simulink library "HORTISIM"  (R2021a)
settings: Solver=VariableStepAuto  StartTime=0.0  StopTime=10.0  RelTol=1e-3
undefined symbols (not defined in the file or in its folder): crop_params, heat_ic, heat_p, p_climate, params_fruit, scr_p, substrate_params, tp_tilapia, win_p, x0_climate, x0_crop, x0_fruit, x0_substrate, x0_tank_tilapia
libraries: $bdroot x10
(part 4 of 4)

== system HORTISIM/Horticulture/Models/Crop Grow/Crop Growth/Growth model/Respiration ==
  T_vmean : Inport
  Crop : Inport  Port=2
  MC_gro : Inport  Port=3
  Bus Creator : BusCreator  Inputs=4
  Bus Selector : BusSelector  OutputSignals=Carbon.Cfruit,Relative.Rfruit,Carbon.Cleaf,Relative.Rleaf,Carbon.Cstem,Relative.Rstem
  Bus Selector2 : BusSelector  OutputSignals=MC_buf_fruit,MC_buf_leaf,MC_buf_stem
  Constant : Constant  Value=params.c_fruit_g
  Constant1 : Constant  Value=params.c_leaf_g
  Constant2 : Constant  Value=params.c_stem_g
  Constant3 : Constant  Value=params.c_fruit_m
  Constant4 : Constant  Value=params.c_leaf_m
  Constant5 : Constant  Value=params.c_stem_m
  Product : Product
  Product1 : Product
  Product2 : Product
  Scope : Scope  NumInputPorts=4
  Subsystem : Subsystem
      settings: PortSchema="{\"entries\":[{\"content\":{\"sides\":[{\"content\":{\"connectorIds\":[\"In1\",\"In2\",\"In3\"]},\"type\":\"ConnectorPlacement.EquallySpacedRectSide\",\"uuid\":\"e383cf86-92c2-4a3a-a03f-0f03c9e6b06e\"},{\"content\":{\"connectorIds\":[\"Out1\"],\"side\":\"RIGHT\"},\"type\":\"ConnectorPlacement.EquallySpacedRectSide\",\"uuid\":\"c4c6234d-4969-4652-ba5e-e62d60415ae5\"},{\"content\":{\"connectorIds\":[\"In4\"],\"side\":\"TOP\"},\"type\":\"ConnectorPlacement.EquallySpacedRectSide\",\"uuid\":\"e372fef3-870c-4656-925c-98a7f16866f7\"}]},\"type\":\"ConnectorPlacement.EquallySpacedConnector\",\"uuid\":\"336e0ef1-3fb5-46ea-bbca-17f64dad2455\"}],\"packageUris\":[\"http://schema.mathworks.com/mf0/Connector/R2020b\"],\"version\":\"1.0\"}"
  Subsystem1 : Subsystem
      settings: PortSchema="{\"entries\":[{\"content\":{\"sides\":[{\"content\":{\"connectorIds\":[\"In1\",\"In2\",\"In3\"]},\"type\":\"ConnectorPlacement.EquallySpacedRectSide\",\"uuid\":\"e383cf86-92c2-4a3a-a03f-0f03c9e6b06e\"},{\"content\":{\"connectorIds\":[\"Out1\"],\"side\":\"RIGHT\"},\"type\":\"ConnectorPlacement.EquallySpacedRectSide\",\"uuid\":\"c4c6234d-4969-4652-ba5e-e62d60415ae5\"},{\"content\":{\"connectorIds\":[\"In4\"],\"side\":\"TOP\"},\"type\":\"ConnectorPlacement.EquallySpacedRectSide\",\"uuid\":\"e372fef3-870c-4656-925c-98a7f16866f7\"}]},\"type\":\"ConnectorPlacement.EquallySpacedConnector\",\"uuid\":\"336e0ef1-3fb5-46ea-bbca-17f64dad2455\"}],\"packageUris\":[\"http://schema.mathworks.com/mf0/Connector/R2020b\"],\"version\":\"1.0\"}"
  Subsystem2 : Subsystem
      settings: PortSchema="{\"entries\":[{\"content\":{\"sides\":[{\"content\":{\"connectorIds\":[\"In1\",\"In2\",\"In3\"]},\"type\":\"ConnectorPlacement.EquallySpacedRectSide\",\"uuid\":\"e383cf86-92c2-4a3a-a03f-0f03c9e6b06e\"},{\"content\":{\"connectorIds\":[\"Out1\"],\"side\":\"RIGHT\"},\"type\":\"ConnectorPlacement.EquallySpacedRectSide\",\"uuid\":\"c4c6234d-4969-4652-ba5e-e62d60415ae5\"},{\"content\":{\"connectorIds\":[\"In4\"],\"side\":\"TOP\"},\"type\":\"ConnectorPlacement.EquallySpacedRectSide\",\"uuid\":\"e372fef3-870c-4656-925c-98a7f16866f7\"}]},\"type\":\"ConnectorPlacement.EquallySpacedConnector\",\"uuid\":\"336e0ef1-3fb5-46ea-bbca-17f64dad2455\"}],\"packageUris\":[\"http://schema.mathworks.com/mf0/Connector/R2020b\"],\"version\":\"1.0\"}"
  Sum : Sum  Inputs=|+++
  MC_resp : Outport
  wires:
  Constant5/1 -> Subsystem2/3(c_m)
  Constant4/1 -> Subsystem1/3(c_m)
  [T_v] -> Subsystem2/4(T_vmean)
  [T_v] -> Subsystem1/4(T_vmean)
  [T_v] -> Subsystem/4(T_vmean)
  Constant3/1 -> Subsystem/3(c_m)
  T_vmean/1 -> [T_v]
  Product1/1 -> Sum/3
  Product2/1 -> Sum/2
  Constant1/1 -> Product2/2
  Constant/1 -> Product/2
  Constant2/1 -> Product1/2
  Product/1 -> Sum/1
  Sum/1 -> Scope/1, Bus Creator/1  "MC_buf_i"
  Bus Selector2/3 -> Product1/1  "<MC_buf_stem>"
  Bus Selector2/2 -> Product2/1  "<MC_buf_leaf>"
  Bus Selector2/1 -> Product/1  "<MC_buf_fruit>"
  Bus Creator/1 -> MC_resp/1
  Subsystem/1(MC_fruit_i) -> Scope/4, Bus Creator/2  "MC_fruit_i"
  Subsystem1/1(MC_leaf_i) -> Scope/2, Bus Creator/3  "MC_leaf_i"
  Subsystem2/1(MC_steam_i) -> Scope/3, Bus Creator/4  "MC_stem_i"
  MC_gro/1 -> Bus Selector2/1
  Crop/1 -> Bus Selector/1
  Bus Selector/1 -> Subsystem/1(C)  "<Cfruit>"
  Bus Selector/2 -> Subsystem/2(R)  "<Rfruit>"
  Bus Selector/3 -> Subsystem1/1(C)  "<Cleaf>"
  Bus Selector/4 -> Subsystem1/2(R)  "<Rleaf>"
  Bus Selector/5 -> Subsystem2/1(C)  "<Cstem>"
  Bus Selector/6 -> Subsystem2/2(R)  "<Rstem>"

== system HORTISIM/Horticulture/Models/Crop Grow/Crop Growth/Growth model/Subsystem2 ==
  " " : Inport
  "         " : Inport  Port=2
  Bus Creator : BusCreator  Inputs=5
  Demux : Demux
  "   " : Outport
  wires:
  "         "/1 -> Demux/1
  Demux/2 -> Bus Creator/3  "MC_fruit_i"
  Demux/1 -> Bus Creator/2  "MC_buf_i"
  Demux/3 -> Bus Creator/4  "MC_leaf_i"
  " "/1 -> Bus Creator/1  "MC_i_buf"
  Bus Creator/1 -> "   "/1
  Demux/4 -> Bus Creator/5  "MC_stem_i"

== system HORTISIM/Horticulture/Models/Crop Grow/Merges/Subsystem/Convertion Ratio ==
  Constant : Constant
  Constant1 : Constant  Value=params.fraction_DM
  Divide : Product  Inputs=*/
  Minus : Sum  Inputs=+-
  Out1 : Outport
  wires:
  Minus/1 -> Out1/1
  Constant1/1 -> Divide/2
  Constant/1 -> Divide/1, Minus/2
  Divide/1 -> Minus/1

== system HORTISIM/Horticulture/Models/Substrate Bag/Subsystem3/V0/Subsystem ==
  V : Inport
  Constant : Constant  Value=params.Vmax_subs/3
  Constant1 : Constant  Value=0.5
  Gain : Gain  Gain=500
  Gain3 : Gain  Gain=0.5
  Minus1 : Sum  Inputs=+-
  Product : Product
  Sum1 : Sum  Inputs=|++
  Tanh : Trigonometry  Operator=tanh
  Out1 : Outport
  wires:
  Tanh/1 -> Gain3/1
  Constant1/1 -> Sum1/2
  Gain3/1 -> Sum1/1
  Gain/1 -> Tanh/1
  Constant/1 -> Minus1/2
  V/1 -> Minus1/1
  Minus1/1 -> Product/1, Gain/1
  Sum1/1 -> Product/2
  Product/1 -> Out1/1

== system HORTISIM/Horticulture/Models/Substrate Bag/Subsystem3/V0/Subsystem1 ==
  V : Inport
  Constant1 : Constant  Value=0.5
  Constant2 : Constant  Value=params.Vmin_subs/3
  Gain : Gain  Gain=5e4
  Gain3 : Gain  Gain=0.5
  Minus1 : Sum  Inputs=+-
  Sum1 : Sum  Inputs=|++
  Tanh : Trigonometry  Operator=tanh
  Out1 : Outport
  wires:
  Tanh/1 -> Gain3/1
  Sum1/1 -> Out1/1
  Constant1/1 -> Sum1/2
  Gain3/1 -> Sum1/1
  Gain/1 -> Tanh/1
  Constant2/1 -> Minus1/2
  V/1 -> Minus1/1
  Minus1/1 -> Gain/1

== system HORTISIM/Horticulture/Models/Substrate Bag/Subsystem3/V1/Subsystem ==
  V : Inport
  Constant : Constant  Value=params.Vmax_subs/3
  Constant1 : Constant  Value=0.5
  Gain : Gain  Gain=500
  Gain3 : Gain  Gain=0.5
  Minus1 : Sum  Inputs=+-
  Product : Product
  Sum1 : Sum  Inputs=|++
  Tanh : Trigonometry  Operator=tanh
  Out1 : Outport
  wires:
  Tanh/1 -> Gain3/1
  Constant1/1 -> Sum1/2
  Gain3/1 -> Sum1/1
  Gain/1 -> Tanh/1
  Constant/1 -> Minus1/2
  V/1 -> Minus1/1
  Minus1/1 -> Product/1, Gain/1
  Sum1/1 -> Product/2
  Product/1 -> Out1/1

== system HORTISIM/Horticulture/Models/Substrate Bag/Subsystem3/V1/Subsystem1 ==
  V : Inport
  Constant1 : Constant  Value=0.5
  Constant2 : Constant  Value=params.Vmin_subs/3
  Gain : Gain  Gain=5e4
  Gain3 : Gain  Gain=0.5
  Minus1 : Sum  Inputs=+-
  Sum1 : Sum  Inputs=|++
  Tanh : Trigonometry  Operator=tanh
  Out1 : Outport
  wires:
  Tanh/1 -> Gain3/1
  Sum1/1 -> Out1/1
  Constant1/1 -> Sum1/2
  Gain3/1 -> Sum1/1
  Gain/1 -> Tanh/1
  Constant2/1 -> Minus1/2
  V/1 -> Minus1/1
  Minus1/1 -> Gain/1

== system HORTISIM/Horticulture/Models/Substrate Bag/Subsystem3/V2/Subsystem ==
  V : Inport
  Constant : Constant  Value=params.Vmax_subs/3
  Constant1 : Constant  Value=0.5
  Gain : Gain  Gain=500
  Gain3 : Gain  Gain=0.5
  Minus1 : Sum  Inputs=+-
  Product : Product
  Sum1 : Sum  Inputs=|++
  Tanh : Trigonometry  Operator=tanh
  Out1 : Outport
  wires:
  Tanh/1 -> Gain3/1
  Constant1/1 -> Sum1/2
  Gain3/1 -> Sum1/1
  Gain/1 -> Tanh/1
  Constant/1 -> Minus1/2
  V/1 -> Minus1/1
  Minus1/1 -> Product/1, Gain/1
  Sum1/1 -> Product/2
  Product/1 -> Out1/1

== system HORTISIM/Horticulture/Models/Substrate Bag/Subsystem3/V2/Subsystem1 ==
  V : Inport
  Constant1 : Constant  Value=0.5
  Constant2 : Constant  Value=params.Vmin_subs/3
  Gain : Gain  Gain=5e4
  Gain3 : Gain  Gain=0.5
  Minus1 : Sum  Inputs=+-
  Sum1 : Sum  Inputs=|++
  Tanh : Trigonometry  Operator=tanh
  Out1 : Outport
  wires:
  Tanh/1 -> Gain3/1
  Sum1/1 -> Out1/1
  Constant1/1 -> Sum1/2
  Gain3/1 -> Sum1/1
  Gain/1 -> Tanh/1
  Constant2/1 -> Minus1/2
  V/1 -> Minus1/1
  Minus1/1 -> Gain/1

== system HORTISIM/Aquaculture/Models/Tank Model/Heat Balances/Convection Air 2 Water Tanl Surface/Gr2vG/If Action Subsystem ==
  Gr : Inport
  Action Port : ActionPort
  Constant : Constant  Value=0.25
  Gain : Gain  Gain=0.5
  Pow : Math  Operator=pow  SignedPower=on  RndMeth=Zero  SaturateOnIntegerOverflow=on
  Out1 : Outport
  wires:
  Gr/1 -> Pow/1
  Constant/1 -> Pow/2
  Pow/1 -> Gain/1
  Gain/1 -> Out1/1

== system HORTISIM/Aquaculture/Models/Tank Model/Heat Balances/Convection Air 2 Water Tanl Surface/Gr2vG/If Action Subsystem1 ==
  Gr : Inport
  Action Port : ActionPort
  Constant : Constant  Value=0.25
  Gain : Gain  Gain=0.5
  Pow : Math  Operator=pow  SignedPower=on  RndMeth=Zero  SaturateOnIntegerOverflow=on
  Out1 : Outport
  wires:
  Gain/1 -> Out1/1
  Constant/1 -> Pow/2
  Gr/1 -> Pow/1
  Pow/1 -> Gain/1

== system HORTISIM/Aquaculture/Models/Tank Model/Heat Balances/Convection Air 2 Water Tanl Surface/Re2vR/If Action Subsystem ==
  Re : Inport
  Action Port : ActionPort
  Constant : Constant  Value=0.5
  Gain : Gain  Gain=0.6
  Pow : Math  Operator=pow  SignedPower=on  RndMeth=Zero  SaturateOnIntegerOverflow=on
  Out1 : Outport
  wires:
  Re/1 -> Pow/1
  Constant/1 -> Pow/2
  Pow/1 -> Gain/1
  Gain/1 -> Out1/1

== system HORTISIM/Aquaculture/Models/Tank Model/Heat Balances/Convection Air 2 Water Tanl Surface/Re2vR/If Action Subsystem1 ==
  Re : Inport
  Action Port : ActionPort
  Constant : Constant  Value=0.8
  Gain : Gain  Gain=0.032
  Pow : Math  Operator=pow  SignedPower=on  RndMeth=Zero  SaturateOnIntegerOverflow=on
  Out1 : Outport
  wires:
  Gain/1 -> Out1/1
  Constant/1 -> Pow/2
  Re/1 -> Pow/1
  Pow/1 -> Gain/1

== system HORTISIM/Aquaculture/Models/Tank Model/Heat Balances/Convection Air 2 Water Tanl Surface/Subsystem/If Action Subsystem ==
  In1 : Inport
  In2 : Inport  Port=2
  Action Port : ActionPort
  Out1 : Outport
  Out2 : Outport  Port=2
  wires:
  In1/1 -> Out1/1
  In2/1 -> Out2/1

== system HORTISIM/Aquaculture/Models/Tank Model/Heat Balances/Convection Air 2 Water Tanl Surface/Subsystem/If Action Subsystem1 ==
  In1 : Inport
  In2 : Inport  Port=2
  Action Port : ActionPort
  Out1 : Outport
  Out2 : Outport  Port=2
  wires:
  In1/1 -> Out1/1
  In2/1 -> Out2/1

== system HORTISIM/Aquaculture/Models/Tank Model/Subsystem/Subsystem1/For Each Subsystem/If Action Subsystem ==
  In1 : Inport
  Action Port : ActionPort
  Out1 : Outport
  wires:
  In1/1 -> Out1/1

== system HORTISIM/Aquaculture/Models/Tank Model/Subsystem/Subsystem1/For Each Subsystem/If Action Subsystem1 ==
  X : Inport
  Action Port : ActionPort
  Out1 : Outport
  wires:
  X/1 -> Out1/1

== system HORTISIM/Climate/Models/Climate Model/Gases Exchange/Compute Mid Variables/Subsystem/Ratio of Humidity Sat ==
  <Tair> : Inport
  p_a : Inport  Port=2
  sat_C_w : Inport  Port=3
  " molar mass of water [kg/mol]" : Constant  Value=0.0180
  Divide1 : Product  Inputs=*/
  Divide2 : Product  Inputs=*/
  Gain1 : Gain  Gain=0.62198
  Minus : Sum  Inputs=+-
  Product : Product  Inputs=3
  gas constant [J/mol/K] : Constant  Value=8.3140
  Out1 : Outport
  wires:
  p_a/1 -> Minus/1
  Minus/1 -> Divide2/2
  Gain1/1 -> Out1/1
  sat_C_w/1 -> Product/3
  <Tair>/1 -> Product/1
  Product/1 -> Divide1/1
  " molar mass of water [kg/mol]"/1 -> Divide1/2
  gas constant [J/mol/K]/1 -> Product/2
  Divide1/1 -> Divide2/1, Minus/2  "p_w^*"
  Divide2/1 -> Gain1/1

== system HORTISIM/Horticulture/Models/Crop Grow/Crop Growth/Growth model/Respiration/Subsystem ==
  C : Inport
  R : Inport  Port=2
  c_m : Inport  Port=3
  T_vmean : Inport  Port=4
  Exponetial Term : Subsystem
  Gain : Gain  Gain=0.1
  Minus : Sum  Inputs=+-
  Power : Math  Operator=pow  SaturateOnIntegerOverflow=on
  Product2 : Product  Inputs=4
  Q_10 : Constant  Value=2
  T_25 : Constant  Value=298.1500
  MC_fruit_i : Outport
  wires:
  Product2/1 -> MC_fruit_i/1
  C/1 -> Product2/4
  c_m/1 -> Product2/3
  Power/1 -> Product2/2
  Q_10/1 -> Power/1
  Exponetial Term/1(Out1) -> Product2/1
  R/1 -> Exponetial Term/1(In1)
  Gain/1 -> Power/2
  Minus/1 -> Gain/1
  T_25/1 -> Minus/2
  T_vmean/1 -> Minus/1

== system HORTISIM/Horticulture/Models/Crop Grow/Crop Growth/Growth model/Respiration/Subsystem1 ==
  C : Inport
  R : Inport  Port=2
  c_m : Inport  Port=3
  T_vmean : Inport  Port=4
  Exponetial Term : Subsystem
  Gain : Gain  Gain=0.1
  Minus : Sum  Inputs=+-
  Power : Math  Operator=pow  SaturateOnIntegerOverflow=on
  Product2 : Product  Inputs=4
  Q_10 : Constant  Value=2
  T_25 : Constant  Value=298.1500
  MC_leaf_i : Outport
  wires:
  Product2/1 -> MC_leaf_i/1
  C/1 -> Product2/4
  c_m/1 -> Product2/3
  Power/1 -> Product2/2
  Q_10/1 -> Power/1
  Exponetial Term/1(Out1) -> Product2/1
  R/1 -> Exponetial Term/1(In1)
  Gain/1 -> Power/2
  Minus/1 -> Gain/1
  T_25/1 -> Minus/2
  T_vmean/1 -> Minus/1

== system HORTISIM/Horticulture/Models/Crop Grow/Crop Growth/Growth model/Respiration/Subsystem2 ==
  C : Inport
  R : Inport  Port=2
  c_m : Inport  Port=3
  T_vmean : Inport  Port=4
  Exponetial Term : Subsystem
  Gain : Gain  Gain=0.1
  Minus : Sum  Inputs=+-
  Power : Math  Operator=pow  SaturateOnIntegerOverflow=on
  Product2 : Product  Inputs=4
  Q_10 : Constant  Value=2
  T_25 : Constant  Value=298.1500
  MC_steam_i : Outport
  wires:
  Product2/1 -> MC_steam_i/1
  C/1 -> Product2/4
  c_m/1 -> Product2/3
  Power/1 -> Product2/2
  Q_10/1 -> Power/1
  Exponetial Term/1(Out1) -> Product2/1
  R/1 -> Exponetial Term/1(In1)
  Gain/1 -> Power/2
  Minus/1 -> Gain/1
  T_25/1 -> Minus/2
  T_vmean/1 -> Minus/1

== system HORTISIM/Horticulture/Models/Crop Grow/Crop Growth/Growth model/Respiration/Subsystem/Exponetial Term ==
  In1 : Inport
  Constant : Constant
  Exp : Math  SaturateOnIntegerOverflow=on
  Gain1 : Gain  Gain=-1
  Minus1 : Sum  Inputs=+-
  Product1 : Product
  regression coefficient in maintenance respiration function [s] : Constant  Value=2850000
  Out1 : Outport
  wires:
  Product1/1 -> Gain1/1
  Constant/1 -> Minus1/1
  Gain1/1 -> Exp/1
  Exp/1 -> Minus1/2
  regression coefficient in maintenance respiration function [s]/1 -> Product1/2
  Minus1/1 -> Out1/1
  In1/1 -> Product1/1

== system HORTISIM/Horticulture/Models/Crop Grow/Crop Growth/Growth model/Respiration/Subsystem1/Exponetial Term ==
  In1 : Inport
  Constant : Constant
  Exp : Math  SaturateOnIntegerOverflow=on
  Gain1 : Gain  Gain=-1
  Minus1 : Sum  Inputs=+-
  Product1 : Product
  regression coefficient in maintenance respiration function [s] : Constant  Value=2850000
  Out1 : Outport
  wires:
  Product1/1 -> Gain1/1
  Constant/1 -> Minus1/1
  Gain1/1 -> Exp/1
  Exp/1 -> Minus1/2
  regression coefficient in maintenance respiration function [s]/1 -> Product1/2
  Minus1/1 -> Out1/1
  In1/1 -> Product1/1

== system HORTISIM/Horticulture/Models/Crop Grow/Crop Growth/Growth model/Respiration/Subsystem2/Exponetial Term ==
  In1 : Inport
  Constant : Constant
  Exp : Math  SaturateOnIntegerOverflow=on
  Gain1 : Gain  Gain=-1
  Minus1 : Sum  Inputs=+-
  Product1 : Product
  regression coefficient in maintenance respiration function [s] : Constant  Value=2850000
  Out1 : Outport
  wires:
  Product1/1 -> Gain1/1
  Constant/1 -> Minus1/1
  Gain1/1 -> Exp/1
  Exp/1 -> Minus1/2
  regression coefficient in maintenance respiration function [s]/1 -> Product1/2
  Minus1/1 -> Out1/1
  In1/1 -> Product1/1

== matlab function HORTISIM/Climate/Models/Climate Model/Indoor Temperature Model/Conduction/Conduction ==
  data: T_f input; T_s1 input; QD_sf1 output; QD_s12 output; A_f input; lam_s input; l_s input; T_ss input
function [QD_sf1,QD_s12] = fcn(T_f,T_s1,A_f,lam_s,l_s,T_ss)

%
%%
% GEOMETRY
% ========
% A_f = p.A_f; % greenhouse floor area [m^2]
% 
% % FLOOR 
% % =====================
% lam_s= p.lam_s; %thermal conductivity of soil layers [W/mK] Concrete, Soil, Clay
% l_s  = p.l_s; %thickness of soil layers [m]
% 
% T_ss = p.T_ss; %deep soil temperature [K]

%%      Conduction
% Floor layers 
% 
QD_sf1 = A_f*lam_s(1)/l_s(1).*(T_f - T_s1); 
QD_s12 = A_f*lam_s(2)/l_s(2).*(T_s1 - T_ss);

== matlab function HORTISIM/Climate/Models/Climate Model/Indoor Temperature Model/Convection/Convection/Convection ==
  data: QV_c_e output; QV_i_c output; QV_i_f output; T_c input; T_i input; T_f input; T_e input; wind_speed input; QP_i_c output; QP_i_f output; C_w input; rho_i input; A_f input; A_c input; d_c input; d_f input; int_air_speed input; C_w_sat_T_c input; C_w_sat_T_f input
function [QV_c_e,QV_i_c,QV_i_f,QP_i_c,QP_i_f] = fcn( T_c,T_i,T_f,T_e,wind_speed,C_w,rho_i,A_f,A_c,d_c,d_f,int_air_speed,C_w_sat_T_c,C_w_sat_T_f)

% CONSTANTS
% =========
g = 9.8100; % acceleration due to gravity [m/s^2]
lambda = 0.0250; % thermal conductivity of air [W/m/K]

Le = 0.8190; % Lewis number [-] 
nu =  1.5100e-05; % kinematic viscosity [m^2/s]

%%
c_i = 1.0032e+03;
H_fg = 2437000;

%%

if wind_speed<0
    wind_speed = 0;
end
%%      Convection

% The Grashof and Reynolds numbers are calculated, and then the Nusselt
% number calculated as the larger of the 'free' Nusselt number, based on
% the Grashof number, and the 'forced' Nusselt number, based on the
% Reynolds number. The heat transferred per unit time is then calculated
% based on this. The first subscript is where heat is transferred from, and
% the second subscript where heat is transferred to.

% Cover to external air
Gr = g*d_c^3/(T_e*nu^2)*abs(T_c - T_e);
Re = wind_speed*d_c/nu;
Nu = lamorturb(Gr, Re);
QV_c_e = 4*A_c.*Nu*lambda.*(T_c - T_e)/d_c;

% Internal air to cover
Gr = g*d_c^3./(T_i*nu^2).*abs(T_i - T_c);
Re = int_air_speed*d_c/nu;  
[Nu, Sh] = lamorturb(Gr, Re, Le);
QV_i_c = 4*A_c.*Nu*lambda.*(T_i - T_c)/d_c;
QP_i_c = 4*A_c*H_fg./(rho_i*c_i).*Sh/Le*lambda/d_c.*(C_w - C_w_sat_T_c);
%QP_i_c = max(QP_i_c,0); % assumed no evaporation from the cover, only condensation

%Internal air to floor
Gr = g*d_f^3./(T_i*nu^2).*abs(T_i - T_f); 
Re = int_air_speed*d_f/nu;
[Nu, Sh] = lamorturb(Gr, Re, Le);
QV_i_f = A_f.*Nu*lambda.*(T_i - T_f)/d_f;
QP_i_f = A_f*H_fg./(rho_i*c_i).*Sh/Le*lambda/d_f.*(C_w - C_w_sat_T_f); 
%QP_i_f = max(QP_i_f,0); % assumed no evaporation from the floor, only condensation

== matlab function HORTISIM/Horticulture/Models/Fruit Partitioning1/MATLAB Function ==
  data: Cfruit input; dCmdt output; Tsum input; Cfruit_mature input; T input; DT output
function [dCmdt,DT] = fcn(Cfruit, Tsum, Cfruit_mature,T)

a = 0.05;

T = T-273.15;
DT = a*max(0,min(1,0.0714*(T-9)));

dCmdt = (Tsum<2600)*DT*(Tsum>1200)*(Cfruit-Cfruit_mature);

== matlab function HORTISIM/Climate/Models/Climate Model/Indoor Temperature Model/Heat Balance/ Soil ==
  data: QD_sf1 input; QD_s12 input; dT_s1_dt output; A_f input; c_s input; l_s input; rhod_s input
function dT_s1_dt  = fcn(QD_sf1,QD_s12,A_f,c_s,l_s,rhod_s)



%% Soil 1
c_Ts1 = 1./(rhod_s(2) * c_s(2) * l_s(2)*A_f);
%
dT_s1_dt = c_Ts1*(QD_sf1 - QD_s12);
%%

== matlab function HORTISIM/Horticulture/Models/Crop Grow/Air Convection/ Temperature ==
  data: QS_v_VIS input; QT_v_i input; QV_v_i input; dT_v_dt output; A_v input; LAI input; msd_v input
function dT_v_dt  = fcn(QS_v_VIS,QT_v_i,QV_v_i,A_v,LAI,msd_v)

c_v   = 4180; % heat capacity of vegetation [J/kgK]
%msd_v = p.msd_v; % surface density [kg/m^2]
%A_v   = p.A_v;

%% Vegetation Temperature
c_Tv = 1./(c_v* A_v.*LAI.*msd_v);
% 
dT_v_dt = c_Tv*( - QV_v_i  - QT_v_i + QS_v_VIS); 
%% Air Temperature

== matlab function HORTISIM/Horticulture/Models/Crop Grow/Air Convection/Subsystem/Convection1 ==
  data: T_i input; Nu input; T_v input; LAI input; QV_v_i output; A_v input; HV output; d_v input
function [QV_v_i,HV] = fcn(T_i,Nu,T_v,LAI,A_v,d_v)


lambda = 0.250; % thermal conductivity of air [W/m/K]
A_v_exp = LAI*A_v; % Area vegetation exposed
QV_v_i = A_v_exp.*Nu*lambda.*(T_v - T_i)/d_v;
HV = Nu*lambda/d_v; % Used in the transpiration term

== matlab function HORTISIM/Horticulture/Models/Crop Grow/Air Convection/Subsystem/Raynols ==
  data: Nu output; T_i input; T_v input; d_v input; int_air_speed input
 function Nu  = fcn(T_i,T_v,d_v,int_air_speed )


% CONSTANTS
% =========
g =     9.8100; % acceleration due to gravity [m/s^2]
nu = 1.5100e-05; % kinematic viscosity [m^2/s]
% VEGETATION CHARACTERISTICS
% ==========================
%d_v = p.d_v; % characteristic leaf length [m]
%int_air_speed = p.int_air_speed;
%%

%%      Convection
% Vegetation to internal air
Gr = g*d_v^3./(T_i*nu^2).*abs(T_v - T_i);
Re = int_air_speed*d_v/nu;
Nu = lamorturb(Gr, Re);

== matlab function HORTISIM/Horticulture/Models/Crop Grow/Crop Growth/Growth model/Growth Organs/Derivatives ==
  data: MC_i_buf input; dC_buff_dt output; dC_fruit_dt output; dC_leaf_dt output; dC_stem_dt output; MC_buf_fruit input; MC_buf_leaf input; MC_buf_stem input; MC_buff_i input; MC_fruit_i input; MC_leaf_i input; MC_stem_i input; MC_leaf_prune input; harvest input
function [dC_buff_dt,dC_fruit_dt,dC_leaf_dt,dC_stem_dt] = fcn(MC_i_buf,MC_buf_fruit,MC_buf_leaf,MC_buf_stem,MC_buff_i,MC_fruit_i,MC_leaf_i,MC_stem_i,MC_leaf_prune, harvest)
%% CALCULATING DERIVATIVES


dC_buff_dt = MC_i_buf - MC_buf_fruit - MC_buf_leaf - MC_buf_stem - MC_buff_i ;

% Plant carbon exchange
dC_fruit_dt = MC_buf_fruit - MC_fruit_i - harvest;

dC_leaf_dt  = MC_buf_leaf  - MC_leaf_i - MC_leaf_prune;

dC_stem_dt  = MC_buf_stem  - MC_stem_i ;

== matlab function HORTISIM/Horticulture/Models/Crop Grow/Crop Growth/Growth model/Photosynthesis/MATLAB Function ==
  data: T_v input; LAI input; Gamma output
function Gamma = fcn(T_v,LAI)

T_k = 273.1500; % zero celsius [K]
c_Gamma         = 1.7000e-06; % effect of canopy temperature on CO2 compensation point [mol{CO2}/mol{air}/K]

Gamma = (c_Gamma*(T_v - T_k)./LAI + 20*c_Gamma*(1 - 1./LAI)); % The CO2 compensation point [mol{CO2}/mol{air}]

== matlab function HORTISIM/Horticulture/Models/Crop Grow/Crop Growth/Growth model/Photosynthesis/Photosyntesis ==
  data: QS_v_VIS input; MC_i_buf output; LAI input; C_c input; rho_i input; T_v input; Gamma input; A_v input; PAR output; P output; Resp output; C_stom output
   function [MC_i_buf,PAR,P,Resp,C_stom] = fcn(QS_v_VIS,LAI,C_c,rho_i,T_v,Gamma,A_v)

%%
% CONSTANTS
% =========
N_A =    6.0221e+23; % Avogadro's number
M_a = 0.0290; % molar mass of dry air [kg/mol]                                                                 
R =     8.3140; % gas constant [J/mol/K]
M_c = 0.0440; % molar mass of CO2 [kg/mol]
T_25 = 298.1500; % K
%
% PHOTOSYNTHESIS MODEL - VANTHOOR
% ===============================
J_max_25        = 2.1000e-04; % maximum rate of electron transport at 25 C [mol{e}/m^2{leaf}/s]
alph            = 0.3850; % conversion factor from photons to electrons [mol{e}/mol{phot}]
theta_constant  = 0.7000; % degree of curvature of the electron transport rate [-]
S               = 710; % entropy term for J_pot calculation [J/mol/K]
HH              = 220000; % deactivation energy for J_pot calculation [J/mol]
E_j             = 37000; % activation energy for J_pot calculation [J/mol]
heat_phot       = 3.6368e-19; % conversion rate from incident energy to number of photons [num{photons}/J]
eta             = 0.6700; % conversion factor from CO2 in the air to CO2 in the stomata [-]
M_carb          = 0.0300; % molar mass of CH2O [kg/mol]

%%

PAR = QS_v_VIS/heat_phot/N_A./A_v; 
% The number of moles of photosynthetically active photons per unit area of planted floor [mol{phot}/m^2/s]
%J/s/(J/photon)/(photons/mol)/m^2 cf Vanthoor 2.3mumol(photons)/J

C_c_molar=(C_c./rho_i).*(M_a/M_c);

%C_stom = eta*C_c_molar; % Stomatal CO2 concentration [mol{CO2}/mol{air}] 
C_stom = eta*C_c_molar; % Stomatal CO2 concentration [mol{CO2}/mol{air}] 

J_pot = LAI*J_max_25.*exp(E_j*(T_v - T_25)./(R*T_v*T_25)).*...
    (1 + exp((S*T_25 - HH)/(R*T_25)))./(1 + exp((S*T_v - HH)./(R*T_v))); % [mol{e}/m^2{floor}s]
%
J = (J_pot + alph*PAR - sqrt((J_pot + alph*PAR).^2 - 4*theta_constant*J_pot*alph.*PAR))/(2*theta_constant);
%
P = J.*(C_stom - Gamma)./(4*(C_stom + 2*Gamma)); % Photosynthesis rate [mol{CO2}/s]
%
Resp = P.*Gamma./C_stom; % Photorespiration rate
%
MC_i_buf = (M_carb.*(P - Resp)); % The net photosynthesis rate [kg{CH2O}/m^2/s]

== matlab function HORTISIM/Horticulture/Models/Crop Grow/Crop Growth/Growth model/Plant Organogenesis /inhibidores ==
  data: T_vmean input; T_vsum input; s_min_T24 input; s_max_T24 input; T_min_v24 input; T_max_v24 input; h_T_v24 output; h_T_vsum output; g_T_v24 output; T_sum_end input
function [h_T_v24,h_T_vsum,g_T_v24] = growth_diff(T_vmean,T_vsum,s_min_T24,s_max_T24,T_min_v24,T_max_v24,T_sum_end)



T_k = 273.15; % zero celsius [K]
%h_T_v24 = 1./(1 + exp(s_min_T24*((T_vmean-T_k) - T_min_v24)))./(1 + exp(s_max_T24*((T_vmean-T_k) - T_max_v24))); 

%k = 0.02;
%h_T_vsum = 0.5 + 0.5*tanh(k*(T_vsum - T_v_start_fruit));

g_T_v24 = 0.047*(T_vmean - T_k) + 0.06;




h_T_v24 = 1./(1 + exp(s_min_T24*((T_vmean-T_k) - T_min_v24)))./(1 + exp(s_max_T24*((T_vmean-T_k) - T_max_v24))); 

h_T_vsum = 0.5*(T_vsum./T_sum_end + sqrt((T_vsum./T_sum_end).^2 + 1e-4)) ...
    - 0.5*(((T_vsum - T_sum_end)/T_sum_end)+sqrt(((T_vsum - T_sum_end)/T_sum_end).^2 + 1e-4)); 


end

== matlab function HORTISIM/Aquaculture/Models/Tank Model/Heat Balances/Transpiration/Ratio of Humidity Sat/MATLAB Function ==
  data: T input; r output
function r  = fcn(T)

expo = 77.3450 + 0.0057*T - 7235/T;

r = exp(expo)/T^8.2;

== matlab function HORTISIM/Horticulture/Models/Crop Grow/Crop Growth/Growth model/Plant Organogenesis /inhibidores1 ==
  data: C_buf input; h_buforg_buf output; C_buf_max input; s_buforg_buf input
function h_buforg_buf  = growth_diff(C_buf,C_buf_max,s_buforg_buf)

%C_buf_min = 0.05*C_buf_max;  
%
%x = (C_buf - C_buf_min);
%h_buforg_buf = (x>0)*(1-exp(-x/0.005));

C_buf_min = 0.05*C_buf_max;
h_buforg_buf =1./(1 + exp(s_buforg_buf*(C_buf - C_buf_min)));


end

== matlab function HORTISIM/Horticulture/Models/Crop Grow/Crop Growth/Growth model/Relative Growth/Relative Growth ==
  data: dC_fruit_dt input; dC_leaf_dt input; dC_stem_dt input; C_fruit input; C_leaf input; C_stem input; R_fruit input; R_leaf input; R_stem input; dR_fruit_dt output; dR_leaf_dt output; dR_stem_dt output; MC_leaf_prune input; harvest input
function [dR_fruit_dt,dR_leaf_dt,dR_stem_dt] = fcn(dC_fruit_dt,dC_leaf_dt,dC_stem_dt,C_fruit,C_leaf,C_stem,R_fruit,R_leaf,R_stem,MC_leaf_prune, harvest)



% Plant growth
dR_fruit_dt = ((dC_fruit_dt + harvest)./C_fruit - R_fruit);
dR_leaf_dt = ((dC_leaf_dt + MC_leaf_prune)./C_leaf - R_leaf);
dR_stem_dt = (dC_stem_dt./C_stem - R_stem);

== matlab function HORTISIM/Horticulture/Models/Crop Grow/Transpiration/MATLAB Function1 ==
  data: vpd input; T_v input; HV input; QS_int input; rho_i input; hL_v_i output
function hL_v_i  = fcn(  vpd,T_v,HV,QS_int ,rho_i )

%%
% CONSTANTS
% =========
T_k  =  273.1500;   % zero celsius [K]
c_i  =  1.0032e+03; % heat capacity of humid air [J/kg/K]                        
H_fg =  2437000;    % latent heat of condensation of water [J/kg]
Le   =  0.8190;     % Lewis number [-] 

% VEGETATION CHARACTERISTICS
%%
Heavy_vpd = vpd/1000 < 0.8;
r_i_vpd   = Heavy_vpd.*(1 + 4.3*(vpd/1000).^2) + (1 - Heavy_vpd)*3.8;

r_st      = 82*((QS_int + 4.3)./(QS_int + 0.54)).*(1 + 0.023*(T_v - T_k - 24.5).^2).*r_i_vpd; %[s/m]

hL_v_i = 2*H_fg./(rho_i*c_i).*(Le^(2/3)./HV + r_st./(rho_i*c_i)).^(-1); %

== matlab function HORTISIM/Climate/Controls/CO2 Pump/MATLAB Function ==
  data: hour input; MC_cc_i output
function MC_cc_i = fcn(hour)

added_CO2 = 0.000;
day_hour_c=(hour/24-floor(hour/24))*24;

track=day_hour_c>6 && day_hour_c<20;
Value=added_CO2/3600;

MC_cc_i=Value*track;

== matlab function HORTISIM/Climate/Controls/Windows Controler/Subsystem/Selection  ==
  data: Rad input; Temperature input; y output; Humidity input; Rad_threshold input
function y = fcn(Rad,Temperature,Humidity,Rad_threshold)

h = double(Rad > Rad_threshold);

y = h*Temperature + (1-h)*Humidity;

%y = Temperature;

== matlab function HORTISIM/Climate/Controls/Windows Controler/Subsystem/Ventilation by Hight Humidity ==
  data: HRInt input; y output; HRStart input; HRMax input
function y = fcn(HRInt,HRStart,HRMax)

H1 = HRStart;
H2 = HRMax;
 
y = 100*( 1 - (HRInt-H2)/(H1-H2));

== matlab function HORTISIM/Climate/Controls/Windows Controler/Subsystem/Ventilation by Hight Temperature1 ==
  data: Tstart input; Ti input; y output; Tmax input
function y = fcn(Tstart,Ti,Tmax)

T1 = Tstart;
T2 = Tmax;

y = 100*( 1 - (Ti-T2)/(T1-T2));

== matlab function HORTISIM/Climate/Models/Climate Model/Indoor Temperature Model/Heat Balance/ Cover ==
  data: QR_c_e input; QS_c input; QV_c_e input; QV_i_c input; QP_i_c input; dT_c_dt output; cd_c input; A_c input
function dT_c_dt = fcn(QR_c_e, QS_c,QV_c_e,QV_i_c,QP_i_c,cd_c,A_c)

%% Cover Temperature
dT_c_dt = 1./(A_c*cd_c).*(+QV_i_c   - QV_c_e  + QS_c + QP_i_c - QR_c_e);

== matlab function HORTISIM/Horticulture/Models/Crop Grow/Crop Growth/Growth model/Plant Organogenesis /inhibidores2 ==
  data: T_v input; s_min_T input; T_min_v input; s_max_T input; T_max_v input; h_T_v output
function h_T_v = growth_diff(T_v,s_min_T,T_min_v,s_max_T,T_max_v)



T_k = 273.15; % zero celsius [K]


h_T_v = 1./(1 + exp(s_min_T*((T_v-T_k) - T_min_v)))./(1 + exp(s_max_T*((T_v-T_k) - T_max_v))); 

end

== matlab function HORTISIM/Climate/Models/Climate Model/Indoor Temperature Model/Heat Balance/ Floor ==
  data: QS_f input; QV_i_f input; QP_i_f input; QD_sf1 input; dT_f_dt output; A_f input; c_s input; l_s input; rhod_s input
function dT_f_dt  = fcn(QS_f,QV_i_f,QP_i_f,QD_sf1,A_f,c_s,l_s,rhod_s)



%% Floor
c_Tf =  1./(rhod_s(1) * A_f * c_s(1) * l_s(1));
%
dT_f_dt  =c_Tf*(QV_i_f  + QS_f - QD_sf1 + QP_i_f);

== matlab function HORTISIM/Climate/Models/Climate Model/Gases Exchange/Compute Mid Variables/Subsystem/Air Density ==
  data: C_w input; C_c input; T_i input; rho_i output; C_c_ppm output; xH output; p_a output
function [rho_i,C_c_ppm,xH,p_a] =   Air(C_w,C_c,T_i)

% CONSTANTS
% =========  
atm = 101300; % standard atmospheric pressure [Pa]
M_a = 0.0290; % molar mass of dry air [kg/mol]                                                                 
R   = 8.3140; % gas constant [J/mol/K]
M_w = 0.0180; % molar mass of water [kg/mol]
M_c = 0.0440; % molar mass of CO2 [kg/mol]


%%
p_w = C_w*R.*T_i/M_w; % Partial pressure of water [Pa]
p_a = (atm - p_w);
rho_i  = (p_a*M_a + p_w*M_w)./(R*T_i); % Density of air [kg/m^3]
C_c_ppm = C_c*R.*T_i/(M_c*atm)*1e6; % CO2 concentration in ppm

xH = 0.62198* p_w /(p_a - p_w);
%%

== matlab function HORTISIM/Climate/Models/Climate Model/Indoor Temperature Model/Heat Balance/ Temperature ==
  data: nu input; rho_i input; QS_i input; QT_fog input; QV_i_e input; QV_i_c input; QV_i input; QV_i_f input; dT_i_dt output; c_i input; V input
function dT_i_dt  = fcn( nu, rho_i ,QS_i,QT_fog,QV_i_e,QV_i_c,QV_i,QV_i_f,c_i,V)


%% Air Temperature

c_Ti = 1./(nu*V.*rho_i*c_i);

dT_i_dt = c_Ti*(  QV_i - QV_i_f - QV_i_c - QV_i_e + QS_i  - QT_fog); 
%%
